simulink model "CRITIS_1_full"  (R2022b)
settings: Solver=VariableStepAuto  StartTime=0.0  StopTime=7  RelTol=1e-3
(part 12 of 13)

== system CRITIS_1_full/TELCOMMUNICATIONS1/delay ==
  in : Inport
  Clock : Clock
  Constant17 : Constant  Value=output
  Switch : Switch  Criteria=u2 > Threshold  Threshold=delay  SaturateOnIntegerOverflow=off  InputSameDT=off
  out : Outport
  wires:
  Switch/1 -> out/1
  Constant17/1 -> Switch/3
  in/1 -> Switch/1
  Clock/1 -> Switch/2

== system CRITIS_1_full/TELCOMMUNICATIONS1/delay1 ==
  in : Inport
  Clock : Clock
  Constant17 : Constant  Value=output
  Switch : Switch  Criteria=u2 > Threshold  Threshold=delay  SaturateOnIntegerOverflow=off  InputSameDT=off
  out : Outport
  wires:
  Switch/1 -> out/1
  Constant17/1 -> Switch/3
  in/1 -> Switch/1
  Clock/1 -> Switch/2

== system CRITIS_1_full/TELCOMMUNICATIONS2/Subsystem1 ==
  servizio : Inport
  Constant : Constant  Value=operation1
  Constant2 : Constant  Value=consumed1
  Constant6 : Constant  Value=operation2
  Constant7 : Constant  Value=num_serv
  Constant9 : Constant  Value=out_service
  Display : Display
  Display1 : Display
  MATLAB Function2 : MATLAB Function  TreatAsAtomicUnit=on
  EXT : Outport
  EXT_V : Outport  Port=2
  wires:
  Constant7/1 -> MATLAB Function2/5(num_serv)
  Constant9/1 -> MATLAB Function2/6(out_service)
  servizio/1 -> MATLAB Function2/1(servizio)
  Constant/1 -> Display/1, MATLAB Function2/3(operation1)
  Constant6/1 -> Display1/1, MATLAB Function2/4(operation2)
  MATLAB Function2/1(se) -> EXT/1
  MATLAB Function2/2(se_vect) -> EXT_V/1
  Constant2/1 -> MATLAB Function2/2(consumed)

== system CRITIS_1_full/TELCOMMUNICATIONS2/Subsystem3 ==
  servizio : Inport
  Constant : Constant  Value=operation1
  Constant2 : Constant  Value=consumed1
  Constant6 : Constant  Value=operation2
  Constant7 : Constant  Value=num_serv
  Constant9 : Constant  Value=out_service
  Display : Display
  Display1 : Display
  MATLAB Function2 : MATLAB Function  TreatAsAtomicUnit=on
  EXT : Outport
  EXT_V : Outport  Port=2
  wires:
  Constant7/1 -> MATLAB Function2/5(num_serv)
  Constant9/1 -> MATLAB Function2/6(out_service)
  servizio/1 -> MATLAB Function2/1(servizio)
  Constant/1 -> Display/1, MATLAB Function2/3(operation1)
  Constant6/1 -> Display1/1, MATLAB Function2/4(operation2)
  MATLAB Function2/1(se) -> EXT/1
  MATLAB Function2/2(se_vect) -> EXT_V/1
  Constant2/1 -> MATLAB Function2/2(consumed)

== system CRITIS_1_full/TELCOMMUNICATIONS2/Subsystem5 ==
  servizio : Inport
  Constant : Constant  Value=operation1
  Constant2 : Constant  Value=consumed1
  Constant6 : Constant  Value=operation2
  Constant7 : Constant  Value=num_serv
  Constant9 : Constant  Value=out_service
  Display : Display
  Display1 : Display
  MATLAB Function2 : MATLAB Function  TreatAsAtomicUnit=on
  EXT : Outport
  EXT_V : Outport  Port=2
  wires:
  Constant7/1 -> MATLAB Function2/5(num_serv)
  Constant9/1 -> MATLAB Function2/6(out_service)
  servizio/1 -> MATLAB Function2/1(servizio)
  Constant/1 -> Display/1, MATLAB Function2/3(operation1)
  Constant6/1 -> Display1/1, MATLAB Function2/4(operation2)
  MATLAB Function2/1(se) -> EXT/1
  MATLAB Function2/2(se_vect) -> EXT_V/1
  Constant2/1 -> MATLAB Function2/2(consumed)

== system CRITIS_1_full/TELCOMMUNICATIONS2/Subsystem6 ==
  servizio : Inport
  Constant : Constant  Value=operation1
  Constant2 : Constant  Value=consumed1
  Constant6 : Constant  Value=operation2
  Constant7 : Constant  Value=num_serv
  Constant9 : Constant  Value=out_service
  MATLAB Function2 : MATLAB Function  TreatAsAtomicUnit=on
  EXT : Outport
  EXT_V : Outport  Port=2
  wires:
  Constant7/1 -> MATLAB Function2/5(num_serv)
  Constant9/1 -> MATLAB Function2/6(out_service)
  servizio/1 -> MATLAB Function2/1(servizio)
  Constant/1 -> MATLAB Function2/3(operation1)
  Constant6/1 -> MATLAB Function2/4(operation2)
  MATLAB Function2/1(se) -> EXT/1
  MATLAB Function2/2(se_vect) -> EXT_V/1
  Constant2/1 -> MATLAB Function2/2(consumed)

== system CRITIS_1_full/TELCOMMUNICATIONS2/Subsystem7 ==
  servizio : Inport
  Constant : Constant  Value=operation1
  Constant2 : Constant  Value=consumed1
  Constant6 : Constant  Value=operation2
  Constant7 : Constant  Value=num_serv
  Constant9 : Constant  Value=out_service
  MATLAB Function2 : MATLAB Function  TreatAsAtomicUnit=on
  EXT : Outport
  EXT_V : Outport  Port=2
  wires:
  Constant7/1 -> MATLAB Function2/5(num_serv)
  Constant9/1 -> MATLAB Function2/6(out_service)
  servizio/1 -> MATLAB Function2/1(servizio)
  Constant/1 -> MATLAB Function2/3(operation1)
  Constant6/1 -> MATLAB Function2/4(operation2)
  MATLAB Function2/1(se) -> EXT/1
  MATLAB Function2/2(se_vect) -> EXT_V/1
  Constant2/1 -> MATLAB Function2/2(consumed)

== system CRITIS_1_full/TELCOMMUNICATIONS2/delay ==
  in : Inport
  Clock : Clock
  Constant17 : Constant  Value=output
  Switch : Switch  Criteria=u2 > Threshold  Threshold=delay  SaturateOnIntegerOverflow=off  InputSameDT=off
  out : Outport
  wires:
  Switch/1 -> out/1
  Constant17/1 -> Switch/3
  in/1 -> Switch/1
  Clock/1 -> Switch/2

== system CRITIS_1_full/TELCOMMUNICATIONS2/delay1 ==
  in : Inport
  Clock : Clock
  Constant17 : Constant  Value=output
  Switch : Switch  Criteria=u2 > Threshold  Threshold=delay  SaturateOnIntegerOverflow=off  InputSameDT=off
  out : Outport
  wires:
  Switch/1 -> out/1
  Constant17/1 -> Switch/3
  in/1 -> Switch/1
  Clock/1 -> Switch/2

== matlab function CRITIS_1_full/AIR TRANSPORTATION/ADR_Physical ==
  data: N1 input; Physical output; N2 input
function Physical = f(N1,N2)

Physical = min([N1 N2]);

== matlab function CRITIS_1_full/BANK 1/BANK1_Physical ==
  data: N1 input; Physical output
function Physical = f(N1)

Physical = min([N1]);

== matlab function CRITIS_1_full/TELCOMMUNICATIONS2/Subsystem6/MATLAB Function2 ==
  data: se output double size=1; se_vect output; servizio input; consumed input; operation1 input; operation2 input; num_serv input; out_service input; Service_Fault output
function [se,se_vect,Service_Fault] = Dep(servizio,consumed,operation1,operation2,num_serv,out_service)

Service_Fault=zeros(1,5);

for i=1:num_serv

    if operation1==1 % AND
        
        Service_Fault(i)=max(abs(consumed(:,i).*servizio(:,i)-consumed(:,i)));
      
    else % OR
        
        Service_Fault(i)=1-max(abs(consumed(:,i).*servizio(:,i)));
    end
    
end


se=1-Service_Fault(1);

if num_serv>1
    for i=2:num_serv

      if operation2==1 % AND
        se=min(se,1-Service_Fault(i));
      else % OR
        se=max(se,1-Service_Fault(i));
      end

    end
end

se_vect=zeros(1,20);
if out_service>1
    se_vect(out_service-1)=se;
end

== matlab function CRITIS_1_full/TELCOMMUNICATIONS2/Subsystem7/MATLAB Function2 ==
  data: se output double size=1; se_vect output; servizio input; consumed input; operation1 input; operation2 input; num_serv input; out_service input; Service_Fault output
function [se,se_vect,Service_Fault] = Dep(servizio,consumed,operation1,operation2,num_serv,out_service)

Service_Fault=zeros(1,5);

for i=1:num_serv

    if operation1==1 % AND
        
        Service_Fault(i)=max(abs(consumed(:,i).*servizio(:,i)-consumed(:,i)));
      
    else % OR
        
        Service_Fault(i)=1-max(abs(consumed(:,i).*servizio(:,i)));
    end
    
end


se=1-Service_Fault(1);

if num_serv>1
    for i=2:num_serv

      if operation2==1 % AND
        se=min(se,1-Service_Fault(i));
      else % OR
        se=max(se,1-Service_Fault(i));
      end

    end
end

se_vect=zeros(1,20);
if out_service>1
    se_vect(out_service-1)=se;
end

== matlab function CRITIS_1_full/ENERGY PROVIDER 1/Subsystem3/MATLAB Function2 ==
  data: se output double size=1; se_vect output; servizio input; consumed input; operation1 input; operation2 input; num_serv input; out_service input
function [se,se_vect] = Dep(servizio,consumed,operation1,operation2,num_serv,out_service)

Service_Fault=zeros(1,5);

for i=1:num_serv

    if operation1==1 % AND
        
        Service_Fault(i)=max(abs(consumed(i,:).*servizio(i,:)-consumed(i,:)));
    else % OR
        
        Service_Fault(i)=1-max(abs(consumed(i,:).*servizio(i,:)));
    end
    
end


se=1-Service_Fault(1);

if num_serv>1
    for i=2:num_serv

      if operation2==1 % AND
        se=min(se,1-Service_Fault(i));
      else % OR
        se=max(se,1-Service_Fault(i));
      end

    end
end

se_vect=zeros(1,20);
if out_service>1
    se_vect(out_service-1)=se;
end

== matlab function CRITIS_1_full/TELCOMMUNICATIONS1/Subsystem3/MATLAB Function2 ==
  data: se output double size=1; se_vect output; servizio input; consumed input; operation1 input; operation2 input; num_serv input; out_service input
function [se,se_vect] = Dep(servizio,consumed,operation1,operation2,num_serv,out_service)

Service_Fault=zeros(1,5);

for i=1:num_serv

    if operation1==1 % AND
        
        Service_Fault(i)=max(abs(consumed(i,:).*servizio(i,:)-consumed(i,:)));
    else % OR
        
        Service_Fault(i)=1-max(abs(consumed(i,:).*servizio(i,:)));
    end
    
end


se=1-Service_Fault(1);

if num_serv>1
    for i=2:num_serv

      if operation2==1 % AND
        se=min(se,1-Service_Fault(i));
      else % OR
        se=max(se,1-Service_Fault(i));
      end

    end
end

se_vect=zeros(1,20);
if out_service>1
    se_vect(out_service-1)=se;
end

== matlab function CRITIS_1_full/TELCOMMUNICATIONS1/Subsystem1/MATLAB Function2 ==
  data: se output double size=1; se_vect output; servizio input; consumed input; operation1 input; operation2 input; num_serv input; out_service input
function [se,se_vect] = Dep(servizio,consumed,operation1,operation2,num_serv,out_service)

Service_Fault=zeros(1,5);

for i=1:num_serv

    if operation1==1 % AND
        
        Service_Fault(i)=max(abs(consumed(i,:).*servizio(i,:)-consumed(i,:)));
    else % OR
        
        Service_Fault(i)=1-max(abs(consumed(i,:).*servizio(i,:)));
    end
    
end


se=1-Service_Fault(1);

if num_serv>1
    for i=2:num_serv

      if operation2==1 % AND
        se=min(se,1-Service_Fault(i));
      else % OR
        se=max(se,1-Service_Fault(i));
      end

    end
end

se_vect=zeros(1,20);
if out_service>1
    se_vect(out_service-1)=se;
end

== matlab function CRITIS_1_full/TELCOMMUNICATIONS1/Subsystem5/MATLAB Function2 ==
  data: se output double size=1; se_vect output; servizio input; consumed input; operation1 input; operation2 input; num_serv input; out_service input
function [se,se_vect] = Dep(servizio,consumed,operation1,operation2,num_serv,out_service)

Service_Fault=zeros(1,5);

for i=1:num_serv

    if operation1==1 % AND
        
        Service_Fault(i)=max(abs(consumed(i,:).*servizio(i,:)-consumed(i,:)));
    else % OR
        
        Service_Fault(i)=1-max(abs(consumed(i,:).*servizio(i,:)));
    end
    
end


se=1-Service_Fault(1);

if num_serv>1
    for i=2:num_serv

      if operation2==1 % AND
        se=min(se,1-Service_Fault(i));
      else % OR
        se=max(se,1-Service_Fault(i));
      end

    end
end

se_vect=zeros(1,20);
if out_service>1
    se_vect(out_service-1)=se;
end

== matlab function CRITIS_1_full/ENERGY PROVIDER 2/Subsystem9/MATLAB Function2 ==
  data: se output double size=1; se_vect output; servizio input; consumed input; operation1 input; operation2 input; num_serv input; out_service input; Service_Fault output
function [se,se_vect,Service_Fault] = Dep(servizio,consumed,operation1,operation2,num_serv,out_service)

Service_Fault=zeros(1,5);

for i=1:num_serv

    if operation1==1 % AND
        
        Service_Fault(i)=max(abs(consumed(:,i).*servizio(:,i)-consumed(:,i)));
      
    else % OR
        
        Service_Fault(i)=1-max(abs(consumed(:,i).*servizio(:,i)));
    end
    
end


se=1-Service_Fault(1);

if num_serv>1
    for i=2:num_serv

      if operation2==1 % AND
        se=min(se,1-Service_Fault(i));
      else % OR
        se=max(se,1-Service_Fault(i));
      end

    end
end

se_vect=zeros(1,20);
if out_service>1
    se_vect(out_service-1)=se;
end

== matlab function CRITIS_1_full/TELCOMMUNICATIONS1/Subsystem10/MATLAB Function2 ==
  data: se output double size=1; se_vect output; servizio input; consumed input; operation1 input; operation2 input; num_serv input; out_service input; Service_Fault output
function [se,se_vect,Service_Fault] = Dep(servizio,consumed,operation1,operation2,num_serv,out_service)

Service_Fault=zeros(1,5);

for i=1:num_serv

    if operation1==1 % AND
        
        Service_Fault(i)=max(abs(consumed(:,i).*servizio(:,i)-consumed(:,i)));
      
    else % OR
        
        Service_Fault(i)=1-max(abs(consumed(:,i).*servizio(:,i)));
    end
    
end


se=1-Service_Fault(1);

if num_serv>1
    for i=2:num_serv

      if operation2==1 % AND
        se=min(se,1-Service_Fault(i));
      else % OR
        se=max(se,1-Service_Fault(i));
      end

    end
end

se_vect=zeros(1,20);
if out_service>1
    se_vect(out_service-1)=se;
end

== matlab function CRITIS_1_full/AIR TRANSPORTATION/Subsystem10/MATLAB Function2 ==
  data: se output double size=1; se_vect output; servizio input; consumed input; operation1 input; operation2 input; num_serv input; out_service input; Service_Fault output
function [se,se_vect,Service_Fault] = Dep(servizio,consumed,operation1,operation2,num_serv,out_service)

Service_Fault=zeros(1,5);

for i=1:num_serv

    if operation1==1 % AND
        
        Service_Fault(i)=max(abs(consumed(:,i).*servizio(:,i)-consumed(:,i)));
      
    else % OR
        
        Service_Fault(i)=1-max(abs(consumed(:,i).*servizio(:,i)));
    end
    
end


se=1-Service_Fault(1);

if num_serv>1
    for i=2:num_serv

      if operation2==1 % AND
        se=min(se,1-Service_Fault(i));
      else % OR
        se=max(se,1-Service_Fault(i));
      end

    end
end

se_vect=zeros(1,20);
if out_service>1
    se_vect(out_service-1)=se;
end

== matlab function CRITIS_1_full/ENERGY PROVIDER 2/Subsystem1/MATLAB Function2 ==
  data: se output double size=1; se_vect output; servizio input; consumed input; operation1 input; operation2 input; num_serv input; out_service input; Service_Fault output
function [se,se_vect,Service_Fault] = Dep(servizio,consumed,operation1,operation2,num_serv,out_service)

Service_Fault=zeros(1,5);

for i=1:num_serv

    if operation1==1 % AND
        
        Service_Fault(i)=max(abs(consumed(:,i).*servizio(:,i)-consumed(:,i)));
      
    else % OR
        
        Service_Fault(i)=1-max(abs(consumed(:,i).*servizio(:,i)));
    end
    
end


se=1-Service_Fault(1);

if num_serv>1
    for i=2:num_serv

      if operation2==1 % AND
        se=min(se,1-Service_Fault(i));
      else % OR
        se=max(se,1-Service_Fault(i));
      end

    end
end

se_vect=zeros(1,20);
if out_service>1
    se_vect(out_service-1)=se;
end

== matlab function CRITIS_1_full/mean 1 ==
  data: u input; y output
function y = fcn(u)

y=[0 0];
n=length(u)/2;
y(1) = sum(u(1:2:end))/n;
y(2) = sum(u(2:2:end))/n;

== matlab function CRITIS_1_full/ENERGY PROVIDER 2/Subsystem2/MATLAB Function2 ==
  data: se output double size=1; se_vect output; servizio input; consumed input; operation1 input; operation2 input; num_serv input; out_service input; Service_Fault output
function [se,se_vect,Service_Fault] = Dep(servizio,consumed,operation1,operation2,num_serv,out_service)

Service_Fault=zeros(1,5);

for i=1:num_serv

    if operation1==1 % AND
        
        Service_Fault(i)=max(abs(consumed(:,i).*servizio(:,i)-consumed(:,i)));
      
    else % OR
        
        Service_Fault(i)=1-max(abs(consumed(:,i).*servizio(:,i)));
    end
    
end


se=1-Service_Fault(1);

if num_serv>1
    for i=2:num_serv

      if operation2==1 % AND
        se=min(se,1-Service_Fault(i));
      else % OR
        se=max(se,1-Service_Fault(i));
      end

    end
end

se_vect=zeros(1,20);
if out_service>1
    se_vect(out_service-1)=se;
end

== matlab function CRITIS_1_full/ENERGY PROVIDER 2/Subsystem4/MATLAB Function2 ==
  data: se output double size=1; se_vect output; servizio input; consumed input; operation1 input; operation2 input; num_serv input; out_service input; Service_Fault output
function [se,se_vect,Service_Fault] = Dep(servizio,consumed,operation1,operation2,num_serv,out_service)

Service_Fault=zeros(1,5);

for i=1:num_serv

    if operation1==1 % AND
        
        Service_Fault(i)=max(abs(consumed(:,i).*servizio(:,i)-consumed(:,i)));
      
    else % OR
        
        Service_Fault(i)=1-max(abs(consumed(:,i).*servizio(:,i)));
    end
    
end


se=1-Service_Fault(1);

if num_serv>1
    for i=2:num_serv

      if operation2==1 % AND
        se=min(se,1-Service_Fault(i));
      else % OR
        se=max(se,1-Service_Fault(i));
      end

    end
end

se_vect=zeros(1,20);
if out_service>1
    se_vect(out_service-1)=se;
end

== matlab function CRITIS_1_full/AIR TRANSPORTATION/Subsystem3/MATLAB Function2 ==
  data: se output double size=1; se_vect output; servizio input; consumed input; operation1 input; operation2 input; num_serv input; out_service input
function [se,se_vect] = Dep(servizio,consumed,operation1,operation2,num_serv,out_service)

Service_Fault=zeros(1,5);

for i=1:num_serv

    if operation1==1 % AND
        
        Service_Fault(i)=max(abs(consumed(i,:).*servizio(i,:)-consumed(i,:)));
    else % OR
        
        Service_Fault(i)=1-max(abs(consumed(i,:).*servizio(i,:)));
    end
    
end


se=1-Service_Fault(1);

if num_serv>1
    for i=2:num_serv

      if operation2==1 % AND
        se=min(se,1-Service_Fault(i));
      else % OR
        se=max(se,1-Service_Fault(i));
      end

    end
end

se_vect=zeros(1,20);
if out_service>1
    se_vect(out_service-1)=se;
end

== matlab function CRITIS_1_full/AIR TRANSPORTATION/Subsystem1/MATLAB Function2 ==
  data: se output double size=1; se_vect output; servizio input; consumed input; operation1 input; operation2 input; num_serv input; out_service input
function [se,se_vect] = Dep(servizio,consumed,operation1,operation2,num_serv,out_service)

Service_Fault=zeros(1,5);

for i=1:num_serv

    if operation1==1 % AND
        
        Service_Fault(i)=max(abs(consumed(i,:).*servizio(i,:)-consumed(i,:)));
    else % OR
        
        Service_Fault(i)=1-max(abs(consumed(i,:).*servizio(i,:)));
    end
    
end


se=1-Service_Fault(1);

if num_serv>1
    for i=2:num_serv

      if operation2==1 % AND
        se=min(se,1-Service_Fault(i));
      else % OR
        se=max(se,1-Service_Fault(i));
      end

    end
end

se_vect=zeros(1,20);
if out_service>1
    se_vect(out_service-1)=se;
end

== matlab function CRITIS_1_full/ENERGY PROVIDER 1/Subsystem10/MATLAB Function2 ==
  data: se output double size=1; se_vect output; servizio input; consumed input; operation1 input; operation2 input; num_serv input; out_service input; Service_Fault output
function [se,se_vect,Service_Fault] = Dep(servizio,consumed,operation1,operation2,num_serv,out_service)

Service_Fault=zeros(1,5);

for i=1:num_serv

    if operation1==1 % AND
        
        Service_Fault(i)=max(abs(consumed(:,i).*servizio(:,i)-consumed(:,i)));
      
    else % OR
        
        Service_Fault(i)=1-max(abs(consumed(:,i).*servizio(:,i)));
    end
    
end


se=1-Service_Fault(1);

if num_serv>1
    for i=2:num_serv

      if operation2==1 % AND
        se=min(se,1-Service_Fault(i));
      else % OR
        se=max(se,1-Service_Fault(i));
      end

    end
end

se_vect=zeros(1,20);
if out_service>1
    se_vect(out_service-1)=se;
end

== matlab function CRITIS_1_full/mean 2 ==
  data: u input; y output
function y = fcn(u)

y=[0 0];
n=length(u)/2;
y(1) = sum(u(1:2:end))/n;
y(2) = sum(u(2:2:end))/n;

== matlab function CRITIS_1_full/AIR TRANSPORTATION/Subsystem4/MATLAB Function2 ==
  data: se output double size=1; se_vect output; servizio input; consumed input; operation1 input; operation2 input; num_serv input; out_service input
function [se,se_vect] = Dep(servizio,consumed,operation1,operation2,num_serv,out_service)

Service_Fault=zeros(1,5);

for i=1:num_serv

    if operation1==1 % AND
        
        Service_Fault(i)=max(abs(consumed(i,:).*servizio(i,:)-consumed(i,:)));
    else % OR
        
        Service_Fault(i)=1-max(abs(consumed(i,:).*servizio(i,:)));
    end
    
end


se=1-Service_Fault(1);

if num_serv>1
    for i=2:num_serv

      if operation2==1 % AND
        se=min(se,1-Service_Fault(i));
      else % OR
        se=max(se,1-Service_Fault(i));
      end

    end
end

se_vect=zeros(1,20);
if out_service>1
    se_vect(out_service-1)=se;
end

== matlab function CRITIS_1_full/AIR TRANSPORTATION/Subsystem5/MATLAB Function2 ==
  data: se output double size=1; se_vect output; servizio input; consumed input; operation1 input; operation2 input; num_serv input; out_service input
function [se,se_vect] = Dep(servizio,consumed,operation1,operation2,num_serv,out_service)

Service_Fault=zeros(1,5);

for i=1:num_serv

    if operation1==1 % AND
        
        Service_Fault(i)=max(abs(consumed(i,:).*servizio(i,:)-consumed(i,:)));
    else % OR
        
        Service_Fault(i)=1-max(abs(consumed(i,:).*servizio(i,:)));
    end
    
end


se=1-Service_Fault(1);

if num_serv>1
    for i=2:num_serv

      if operation2==1 % AND
        se=min(se,1-Service_Fault(i));
      else % OR
        se=max(se,1-Service_Fault(i));
      end

    end
end

se_vect=zeros(1,20);
if out_service>1
    se_vect(out_service-1)=se;
end

== matlab function CRITIS_1_full/AIR TRANSPORTATION/Subsystem6/MATLAB Function2 ==
  data: se output double size=1; se_vect output; servizio input; consumed input; operation1 input; operation2 input; num_serv input; out_service input
function [se,se_vect] = Dep(servizio,consumed,operation1,operation2,num_serv,out_service)

Service_Fault=zeros(1,5);

for i=1:num_serv

    if operation1==1 % AND
        
        Service_Fault(i)=max(abs(consumed(i,:).*servizio(i,:)-consumed(i,:)));
    else % OR
        
        Service_Fault(i)=1-max(abs(consumed(i,:).*servizio(i,:)));
    end
    
end


se=1-Service_Fault(1);

if num_serv>1
    for i=2:num_serv

      if operation2==1 % AND
        se=min(se,1-Service_Fault(i));
      else % OR
        se=max(se,1-Service_Fault(i));
      end

    end
end

se_vect=zeros(1,20);
if out_service>1
    se_vect(out_service-1)=se;
end

== matlab function CRITIS_1_full/AIR TRANSPORTATION/Subsystem7/MATLAB Function2 ==
  data: se output double size=1; se_vect output; servizio input; consumed input; operation1 input; operation2 input; num_serv input; out_service input
function [se,se_vect] = Dep(servizio,consumed,operation1,operation2,num_serv,out_service)

Service_Fault=zeros(1,5);

for i=1:num_serv

    if operation1==1 % AND
        
        Service_Fault(i)=max(abs(consumed(i,:).*servizio(i,:)-consumed(i,:)));
    else % OR
        
        Service_Fault(i)=1-max(abs(consumed(i,:).*servizio(i,:)));
    end
    
end


se=1-Service_Fault(1);

if num_serv>1
    for i=2:num_serv

      if operation2==1 % AND
        se=min(se,1-Service_Fault(i));
      else % OR
        se=max(se,1-Service_Fault(i));
      end

    end
end

se_vect=zeros(1,20);
if out_service>1
    se_vect(out_service-1)=se;
end

== matlab function CRITIS_1_full/AIR TRANSPORTATION/Subsystem8/MATLAB Function2 ==
  data: se output double size=1; se_vect output; servizio input; consumed input; operation1 input; operation2 input; num_serv input; out_service input
function [se,se_vect] = Dep(servizio,consumed,operation1,operation2,num_serv,out_service)

Service_Fault=zeros(1,5);

for i=1:num_serv

    if operation1==1 % AND
        
        Service_Fault(i)=max(abs(consumed(i,:).*servizio(i,:)-consumed(i,:)));
    else % OR
        
        Service_Fault(i)=1-max(abs(consumed(i,:).*servizio(i,:)));
    end
    
end


se=1-Service_Fault(1);

if num_serv>1
    for i=2:num_serv

      if operation2==1 % AND
        se=min(se,1-Service_Fault(i));
      else % OR
        se=max(se,1-Service_Fault(i));
      end

    end
end

se_vect=zeros(1,20);
if out_service>1
    se_vect(out_service-1)=se;
end

== matlab function CRITIS_1_full/mean 3 ==
  data: u input; y output
function y = fcn(u)

y=[0 0];
n=length(u)/2;
y(1) = sum(u(1:2:end))/n;
y(2) = sum(u(2:2:end))/n;

== matlab function CRITIS_1_full/RAILWAYS/Subsystem5/MATLAB Function2 ==
  data: se output double size=1; se_vect output; servizio input; consumed input; operation1 input; operation2 input; num_serv input; out_service input
function [se,se_vect] = Dep(servizio,consumed,operation1,operation2,num_serv,out_service)

Service_Fault=zeros(1,5);

for i=1:num_serv

    if operation1==1 % AND
        
        Service_Fault(i)=max(abs(consumed(i,:).*servizio(i,:)-consumed(i,:)));
    else % OR
        
        Service_Fault(i)=1-max(abs(consumed(i,:).*servizio(i,:)));
    end
    
end


se=1-Service_Fault(1);

if num_serv>1
    for i=2:num_serv

      if operation2==1 % AND
        se=min(se,1-Service_Fault(i));
      else % OR
        se=max(se,1-Service_Fault(i));
      end

    end
end

se_vect=zeros(1,20);
if out_service>1
    se_vect(out_service-1)=se;
end

== matlab function CRITIS_1_full/RAILWAYS/Subsystem6/MATLAB Function2 ==
  data: se output double size=1; se_vect output; servizio input; consumed input; operation1 input; operation2 input; num_serv input; out_service input
function [se,se_vect] = Dep(servizio,consumed,operation1,operation2,num_serv,out_service)

Service_Fault=zeros(1,5);

for i=1:num_serv

    if operation1==1 % AND
        
        Service_Fault(i)=max(abs(consumed(i,:).*servizio(i,:)-consumed(i,:)));
    else % OR
        
        Service_Fault(i)=1-max(abs(consumed(i,:).*servizio(i,:)));
    end
    
end


se=1-Service_Fault(1);

if num_serv>1
    for i=2:num_serv

      if operation2==1 % AND
        se=min(se,1-Service_Fault(i));
      else % OR
        se=max(se,1-Service_Fault(i));
      end

    end
end

se_vect=zeros(1,20);
if out_service>1
    se_vect(out_service-1)=se;
end

== matlab function CRITIS_1_full/RAILWAYS/Subsystem1/MATLAB Function2 ==
  data: se output double size=1; se_vect output; servizio input; consumed input; operation1 input; operation2 input; num_serv input; out_service input
function [se,se_vect] = Dep(servizio,consumed,operation1,operation2,num_serv,out_service)

Service_Fault=zeros(1,5);

for i=1:num_serv

    if operation1==1 % AND
        
        Service_Fault(i)=max(abs(consumed(i,:).*servizio(i,:)-consumed(i,:)));
    else % OR
        
        Service_Fault(i)=1-max(abs(consumed(i,:).*servizio(i,:)));
    end
    
end


se=1-Service_Fault(1);

if num_serv>1
    for i=2:num_serv

      if operation2==1 % AND
        se=min(se,1-Service_Fault(i));
      else % OR
        se=max(se,1-Service_Fault(i));
      end

    end
end

se_vect=zeros(1,20);
if out_service>1
    se_vect(out_service-1)=se;
end

== matlab function CRITIS_1_full/RAILWAYS/Subsystem2/MATLAB Function2 ==
  data: se output double size=1; se_vect output; servizio input; consumed input; operation1 input; operation2 input; num_serv input; out_service input
function [se,se_vect] = Dep(servizio,consumed,operation1,operation2,num_serv,out_service)

Service_Fault=zeros(1,5);

for i=1:num_serv

    if operation1==1 % AND
        
        Service_Fault(i)=max(abs(consumed(i,:).*servizio(i,:)-consumed(i,:)));
    else % OR
        
        Service_Fault(i)=1-max(abs(consumed(i,:).*servizio(i,:)));
    end
    
end


se=1-Service_Fault(1);

if num_serv>1
    for i=2:num_serv

      if operation2==1 % AND
        se=min(se,1-Service_Fault(i));
      else % OR
        se=max(se,1-Service_Fault(i));
      end

    end
end

se_vect=zeros(1,20);
if out_service>1
    se_vect(out_service-1)=se;
end

== matlab function CRITIS_1_full/RAILWAYS/Subsystem3/MATLAB Function2 ==
  data: se output double size=1; se_vect output; servizio input; consumed input; operation1 input; operation2 input; num_serv input; out_service input
function [se,se_vect] = Dep(servizio,consumed,operation1,operation2,num_serv,out_service)

Service_Fault=zeros(1,5);

for i=1:num_serv

    if operation1==1 % AND
        
        Service_Fault(i)=max(abs(consumed(i,:).*servizio(i,:)-consumed(i,:)));
    else % OR
        
        Service_Fault(i)=1-max(abs(consumed(i,:).*servizio(i,:)));
    end
    
end


se=1-Service_Fault(1);

if num_serv>1
    for i=2:num_serv

      if operation2==1 % AND
        se=min(se,1-Service_Fault(i));
      else % OR
        se=max(se,1-Service_Fault(i));
      end

    end
end

se_vect=zeros(1,20);
if out_service>1
    se_vect(out_service-1)=se;
end

== matlab function CRITIS_1_full/RAILWAYS/Subsystem4/MATLAB Function2 ==
  data: se output double size=1; se_vect output; servizio input; consumed input; operation1 input; operation2 input; num_serv input; out_service input
function [se,se_vect] = Dep(servizio,consumed,operation1,operation2,num_serv,out_service)

Service_Fault=zeros(1,5);

for i=1:num_serv

    if operation1==1 % AND
        
        Service_Fault(i)=max(abs(consumed(i,:).*servizio(i,:)-consumed(i,:)));
    else % OR
        
        Service_Fault(i)=1-max(abs(consumed(i,:).*servizio(i,:)));
    end
    
end


se=1-Service_Fault(1);

if num_serv>1
    for i=2:num_serv

      if operation2==1 % AND
        se=min(se,1-Service_Fault(i));
      else % OR
        se=max(se,1-Service_Fault(i));
      end

    end
end

se_vect=zeros(1,20);
if out_service>1
    se_vect(out_service-1)=se;
end

== matlab function CRITIS_1_full/mean 4 ==
  data: u input; y output
function y = fcn(u)

y=[0 0];
n=length(u)/2;
y(1) = sum(u(1:2:end))/n;
y(2) = sum(u(2:2:end))/n;

== matlab function CRITIS_1_full/RAILWAYS/Subsystem7/MATLAB Function2 ==
  data: se output double size=1; se_vect output; servizio input; consumed input; operation1 input; operation2 input; num_serv input; out_service input
function [se,se_vect] = Dep(servizio,consumed,operation1,operation2,num_serv,out_service)

Service_Fault=zeros(1,5);

for i=1:num_serv

    if operation1==1 % AND
        
        Service_Fault(i)=max(abs(consumed(i,:).*servizio(i,:)-consumed(i,:)));
    else % OR
        
        Service_Fault(i)=1-max(abs(consumed(i,:).*servizio(i,:)));
    end
    
end


se=1-Service_Fault(1);

if num_serv>1
    for i=2:num_serv

      if operation2==1 % AND
        se=min(se,1-Service_Fault(i));
      else % OR
        se=max(se,1-Service_Fault(i));
      end

    end
end

se_vect=zeros(1,20);
if out_service>1
    se_vect(out_service-1)=se;
end

== matlab function CRITIS_1_full/RAILWAYS/Subsystem8/MATLAB Function2 ==
  data: se output double size=1; se_vect output; servizio input; consumed input; operation1 input; operation2 input; num_serv input; out_service input
function [se,se_vect] = Dep(servizio,consumed,operation1,operation2,num_serv,out_service)

Service_Fault=zeros(1,5);

for i=1:num_serv

    if operation1==1 % AND
        
        Service_Fault(i)=max(abs(consumed(i,:).*servizio(i,:)-consumed(i,:)));
    else % OR
        
        Service_Fault(i)=1-max(abs(consumed(i,:).*servizio(i,:)));
    end
    
end


se=1-Service_Fault(1);

if num_serv>1
    for i=2:num_serv

      if operation2==1 % AND
        se=min(se,1-Service_Fault(i));
      else % OR
        se=max(se,1-Service_Fault(i));
      end

    end
end

se_vect=zeros(1,20);
if out_service>1
    se_vect(out_service-1)=se;
end

== matlab function CRITIS_1_full/RAILWAYS/Subsystem9/MATLAB Function2 ==
  data: se output double size=1; se_vect output; servizio input; consumed input; operation1 input; operation2 input; num_serv input; out_service input
function [se,se_vect] = Dep(servizio,consumed,operation1,operation2,num_serv,out_service)

Service_Fault=zeros(1,5);

for i=1:num_serv

    if operation1==1 % AND
        
        Service_Fault(i)=max(abs(consumed(i,:).*servizio(i,:)-consumed(i,:)));
    else % OR
        
        Service_Fault(i)=1-max(abs(consumed(i,:).*servizio(i,:)));
    end
    
end


se=1-Service_Fault(1);

if num_serv>1
    for i=2:num_serv

      if operation2==1 % AND
        se=min(se,1-Service_Fault(i));
      else % OR
        se=max(se,1-Service_Fault(i));
      end

    end
end

se_vect=zeros(1,20);
if out_service>1
    se_vect(out_service-1)=se;
end

== matlab function CRITIS_1_full/RAILWAYS/Subsystem10/MATLAB Function2 ==
  data: se output double size=1; se_vect output; servizio input; consumed input; operation1 input; operation2 input; num_serv input; out_service input
function [se,se_vect] = Dep(servizio,consumed,operation1,operation2,num_serv,out_service)

Service_Fault=zeros(1,5);

for i=1:num_serv

    if operation1==1 % AND
        
        Service_Fault(i)=max(abs(consumed(i,:).*servizio(i,:)-consumed(i,:)));
    else % OR
        
        Service_Fault(i)=1-max(abs(consumed(i,:).*servizio(i,:)));
    end
    
end


se=1-Service_Fault(1);

if num_serv>1
    for i=2:num_serv

      if operation2==1 % AND
        se=min(se,1-Service_Fault(i));
      else % OR
        se=max(se,1-Service_Fault(i));
      end

    end
end

se_vect=zeros(1,20);
if out_service>1
    se_vect(out_service-1)=se;
end

== matlab function CRITIS_1_full/DEPARTMENT OF INDUSTRIAL DEVELOPMENT/Subsystem1/MATLAB Function2 ==
  data: se output double size=1; se_vect output; servizio input; consumed input; operation1 input; operation2 input; num_serv input; out_service input
function [se,se_vect] = Dep(servizio,consumed,operation1,operation2,num_serv,out_service)

Service_Fault=zeros(1,5);

for i=1:num_serv

    if operation1==1 % AND
        
        Service_Fault(i)=max(abs(consumed(i,:).*servizio(i,:)-consumed(i,:)));
    else % OR
        
        Service_Fault(i)=1-max(abs(consumed(i,:).*servizio(i,:)));
    end
    
end


se=1-Service_Fault(1);

if num_serv>1
    for i=2:num_serv

      if operation2==1 % AND
        se=min(se,1-Service_Fault(i));
      else % OR
        se=max(se,1-Service_Fault(i));
      end

    end
end

se_vect=zeros(1,20);
if out_service>1
    se_vect(out_service-1)=se;
end

== matlab function CRITIS_1_full/RAILWAYS/RFI_Physical ==
  data: N1 input; Physical output; N2 input
function Physical = f(N1,N2)

Physical = min([N1 N2]);

== matlab function CRITIS_1_full/DEPARTMENT OF INDUSTRIAL DEVELOPMENT/Subsystem2/MATLAB Function2 ==
  data: se output double size=1; se_vect output; servizio input; consumed input; operation1 input; operation2 input; num_serv input; out_service input
function [se,se_vect] = Dep(servizio,consumed,operation1,operation2,num_serv,out_service)

Service_Fault=zeros(1,5);

for i=1:num_serv

    if operation1==1 % AND
        
        Service_Fault(i)=max(abs(consumed(i,:).*servizio(i,:)-consumed(i,:)));
    else % OR
        
        Service_Fault(i)=1-max(abs(consumed(i,:).*servizio(i,:)));
    end
    
end


se=1-Service_Fault(1);

if num_serv>1
    for i=2:num_serv

      if operation2==1 % AND
        se=min(se,1-Service_Fault(i));
      else % OR
        se=max(se,1-Service_Fault(i));
      end

    end
end

se_vect=zeros(1,20);
if out_service>1
    se_vect(out_service-1)=se;
end

== matlab function CRITIS_1_full/DEPARTMENT OF INDUSTRIAL DEVELOPMENT/Subsystem3/MATLAB Function2 ==
  data: se output double size=1; se_vect output; servizio input; consumed input; operation1 input; operation2 input; num_serv input; out_service input
function [se,se_vect] = Dep(servizio,consumed,operation1,operation2,num_serv,out_service)

Service_Fault=zeros(1,5);

for i=1:num_serv

    if operation1==1 % AND
        
        Service_Fault(i)=max(abs(consumed(i,:).*servizio(i,:)-consumed(i,:)));
    else % OR
        
        Service_Fault(i)=1-max(abs(consumed(i,:).*servizio(i,:)));
    end
    
end


se=1-Service_Fault(1);

if num_serv>1
    for i=2:num_serv

      if operation2==1 % AND
        se=min(se,1-Service_Fault(i));
      else % OR
        se=max(se,1-Service_Fault(i));
      end

    end
end

se_vect=zeros(1,20);
if out_service>1
    se_vect(out_service-1)=se;
end

== matlab function CRITIS_1_full/DEPARTMENT OF INDUSTRIAL DEVELOPMENT/Subsystem4/MATLAB Function2 ==
  data: se output double size=1; se_vect output; servizio input; consumed input; operation1 input; operation2 input; num_serv input; out_service input
function [se,se_vect] = Dep(servizio,consumed,operation1,operation2,num_serv,out_service)

Service_Fault=zeros(1,5);

for i=1:num_serv

    if operation1==1 % AND
        
        Service_Fault(i)=max(abs(consumed(i,:).*servizio(i,:)-consumed(i,:)));
    else % OR
        
        Service_Fault(i)=1-max(abs(consumed(i,:).*servizio(i,:)));
    end
    
end


se=1-Service_Fault(1);

if num_serv>1
    for i=2:num_serv

      if operation2==1 % AND
        se=min(se,1-Service_Fault(i));
      else % OR
        se=max(se,1-Service_Fault(i));
      end

    end
end

se_vect=zeros(1,20);
if out_service>1
    se_vect(out_service-1)=se;
end

== matlab function CRITIS_1_full/DEPARTMENT OF INDUSTRIAL DEVELOPMENT/Subsystem5/MATLAB Function2 ==
  data: se output double size=1; se_vect output; servizio input; consumed input; operation1 input; operation2 input; num_serv input; out_service input
function [se,se_vect] = Dep(servizio,consumed,operation1,operation2,num_serv,out_service)

Service_Fault=zeros(1,5);

for i=1:num_serv

    if operation1==1 % AND
        
        Service_Fault(i)=max(abs(consumed(i,:).*servizio(i,:)-consumed(i,:)));
    else % OR
        
        Service_Fault(i)=1-max(abs(consumed(i,:).*servizio(i,:)));
    end
    
end


se=1-Service_Fault(1);

if num_serv>1
    for i=2:num_serv

      if operation2==1 % AND
        se=min(se,1-Service_Fault(i));
      else % OR
        se=max(se,1-Service_Fault(i));
      end

    end
end

se_vect=zeros(1,20);
if out_service>1
    se_vect(out_service-1)=se;
end

== matlab function CRITIS_1_full/DEPARTMENT OF INDUSTRIAL DEVELOPMENT/Subsystem6/MATLAB Function2 ==
  data: se output double size=1; se_vect output; servizio input; consumed input; operation1 input; operation2 input; num_serv input; out_service input
function [se,se_vect] = Dep(servizio,consumed,operation1,operation2,num_serv,out_service)

Service_Fault=zeros(1,5);

for i=1:num_serv

    if operation1==1 % AND
        
        Service_Fault(i)=max(abs(consumed(i,:).*servizio(i,:)-consumed(i,:)));
    else % OR
        
        Service_Fault(i)=1-max(abs(consumed(i,:).*servizio(i,:)));
    end
    
end


se=1-Service_Fault(1);

if num_serv>1
    for i=2:num_serv

      if operation2==1 % AND
        se=min(se,1-Service_Fault(i));
      else % OR
        se=max(se,1-Service_Fault(i));
      end

    end
end

se_vect=zeros(1,20);
if out_service>1
    se_vect(out_service-1)=se;
end

== matlab function CRITIS_1_full/BANK 1/Subsystem1/MATLAB Function2 ==
  data: se output double size=1; se_vect output; servizio input; consumed input; operation1 input; operation2 input; num_serv input; out_service input
function [se,se_vect] = Dep(servizio,consumed,operation1,operation2,num_serv,out_service)

Service_Fault=zeros(1,5);

for i=1:num_serv

    if operation1==1 % AND
        
        Service_Fault(i)=max(abs(consumed(i,:).*servizio(i,:)-consumed(i,:)));
    else % OR
        
        Service_Fault(i)=1-max(abs(consumed(i,:).*servizio(i,:)));
    end
    
end


se=1-Service_Fault(1);

if num_serv>1
    for i=2:num_serv

      if operation2==1 % AND
        se=min(se,1-Service_Fault(i));
      else % OR
        se=max(se,1-Service_Fault(i));
      end

    end
end

se_vect=zeros(1,20);
if out_service>1
    se_vect(out_service-1)=se;
end

== matlab function CRITIS_1_full/ENERGY PROVIDER 2/ARETI_Physical ==
  data: N1 input; Physical output; N2 input; N3 input; N4 input
function Physical = f(N1,N2,N3,N4)

Physical = min([N1 N2 N3 N4]);

== matlab function CRITIS_1_full/BANK 1/Subsystem2/MATLAB Function2 ==
  data: se output double size=1; se_vect output; servizio input; consumed input; operation1 input; operation2 input; num_serv input; out_service input
function [se,se_vect] = Dep(servizio,consumed,operation1,operation2,num_serv,out_service)

Service_Fault=zeros(1,5);

for i=1:num_serv

    if operation1==1 % AND
        
        Service_Fault(i)=max(abs(consumed(i,:).*servizio(i,:)-consumed(i,:)));
    else % OR
        
        Service_Fault(i)=1-max(abs(consumed(i,:).*servizio(i,:)));
    end
    
end


se=1-Service_Fault(1);

if num_serv>1
    for i=2:num_serv

      if operation2==1 % AND
        se=min(se,1-Service_Fault(i));
      else % OR
        se=max(se,1-Service_Fault(i));
      end

    end
end

se_vect=zeros(1,20);
if out_service>1
    se_vect(out_service-1)=se;
end

== matlab function CRITIS_1_full/BANK 1/Subsystem3/MATLAB Function2 ==
  data: se output double size=1; se_vect output; servizio input; consumed input; operation1 input; operation2 input; num_serv input; out_service input
function [se,se_vect] = Dep(servizio,consumed,operation1,operation2,num_serv,out_service)

Service_Fault=zeros(1,5);

for i=1:num_serv

    if operation1==1 % AND
        
        Service_Fault(i)=max(abs(consumed(i,:).*servizio(i,:)-consumed(i,:)));
    else % OR
        
        Service_Fault(i)=1-max(abs(consumed(i,:).*servizio(i,:)));
    end
    
end


se=1-Service_Fault(1);

if num_serv>1
    for i=2:num_serv

      if operation2==1 % AND
        se=min(se,1-Service_Fault(i));
      else % OR
        se=max(se,1-Service_Fault(i));
      end

    end
end

se_vect=zeros(1,20);
if out_service>1
    se_vect(out_service-1)=se;
end

== matlab function CRITIS_1_full/BANK 1/Subsystem4/MATLAB Function2 ==
  data: se output double size=1; se_vect output; servizio input; consumed input; operation1 input; operation2 input; num_serv input; out_service input
function [se,se_vect] = Dep(servizio,consumed,operation1,operation2,num_serv,out_service)

Service_Fault=zeros(1,5);

for i=1:num_serv

    if operation1==1 % AND
        
        Service_Fault(i)=max(abs(consumed(i,:).*servizio(i,:)-consumed(i,:)));
    else % OR
        
        Service_Fault(i)=1-max(abs(consumed(i,:).*servizio(i,:)));
    end
    
end


se=1-Service_Fault(1);

if num_serv>1
    for i=2:num_serv

      if operation2==1 % AND
        se=min(se,1-Service_Fault(i));
      else % OR
        se=max(se,1-Service_Fault(i));
      end

    end
end

se_vect=zeros(1,20);
if out_service>1
    se_vect(out_service-1)=se;
end

== matlab function CRITIS_1_full/BANK 1/Subsystem5/MATLAB Function2 ==
  data: se output double size=1; se_vect output; servizio input; consumed input; operation1 input; operation2 input; num_serv input; out_service input
function [se,se_vect] = Dep(servizio,consumed,operation1,operation2,num_serv,out_service)

Service_Fault=zeros(1,5);

for i=1:num_serv

    if operation1==1 % AND
        
        Service_Fault(i)=max(abs(consumed(i,:).*servizio(i,:)-consumed(i,:)));
    else % OR
        
        Service_Fault(i)=1-max(abs(consumed(i,:).*servizio(i,:)));
    end
    
end


se=1-Service_Fault(1);

if num_serv>1
    for i=2:num_serv

      if operation2==1 % AND
        se=min(se,1-Service_Fault(i));
      else % OR
        se=max(se,1-Service_Fault(i));
      end

    end
end

se_vect=zeros(1,20);
if out_service>1
    se_vect(out_service-1)=se;
end

== matlab function CRITIS_1_full/BANK 1/Subsystem6/MATLAB Function2 ==
  data: se output double size=1; se_vect output; servizio input; consumed input; operation1 input; operation2 input; num_serv input; out_service input
function [se,se_vect] = Dep(servizio,consumed,operation1,operation2,num_serv,out_service)

Service_Fault=zeros(1,5);

for i=1:num_serv

    if operation1==1 % AND
        
        Service_Fault(i)=max(abs(consumed(i,:).*servizio(i,:)-consumed(i,:)));
    else % OR
        
        Service_Fault(i)=1-max(abs(consumed(i,:).*servizio(i,:)));
    end
    
end


se=1-Service_Fault(1);

if num_serv>1
    for i=2:num_serv

      if operation2==1 % AND
        se=min(se,1-Service_Fault(i));
      else % OR
        se=max(se,1-Service_Fault(i));
      end

    end
end

se_vect=zeros(1,20);
if out_service>1
    se_vect(out_service-1)=se;
end

== matlab function CRITIS_1_full/AIR TRANSPORTATION/Subsystem9/MATLAB Function2 ==
  data: se output double size=1; se_vect output; servizio input; consumed input; operation1 input; operation2 input; num_serv input; out_service input; Service_Fault output
function [se,se_vect,Service_Fault] = Dep(servizio,consumed,operation1,operation2,num_serv,out_service)

Service_Fault=zeros(1,5);

for i=1:num_serv

    if operation1==1 % AND
        
        Service_Fault(i)=max(abs(consumed(:,i).*servizio(:,i)-consumed(:,i)));
      
    else % OR
        
        Service_Fault(i)=1-max(abs(consumed(:,i).*servizio(:,i)));
    end
    
end


se=1-Service_Fault(1);

if num_serv>1
    for i=2:num_serv

      if operation2==1 % AND
        se=min(se,1-Service_Fault(i));
      else % OR
        se=max(se,1-Service_Fault(i));
      end

    end
end

se_vect=zeros(1,20);
if out_service>1
    se_vect(out_service-1)=se;
end

== matlab function CRITIS_1_full/RAILWAYS/Subsystem11/MATLAB Function2 ==
  data: se output double size=1; se_vect output; servizio input; consumed input; operation1 input; operation2 input; num_serv input; out_service input; Service_Fault output
function [se,se_vect,Service_Fault] = Dep(servizio,consumed,operation1,operation2,num_serv,out_service)

Service_Fault=zeros(1,5);

for i=1:num_serv

    if operation1==1 % AND
        
        Service_Fault(i)=max(abs(consumed(:,i).*servizio(:,i)-consumed(:,i)));
      
    else % OR
        
        Service_Fault(i)=1-max(abs(consumed(:,i).*servizio(:,i)));
    end
    
end


se=1-Service_Fault(1);

if num_serv>1
    for i=2:num_serv

      if operation2==1 % AND
        se=min(se,1-Service_Fault(i));
      else % OR
        se=max(se,1-Service_Fault(i));
      end

    end
end

se_vect=zeros(1,20);
if out_service>1
    se_vect(out_service-1)=se;
end

== matlab function CRITIS_1_full/TELCOMMUNICATIONS2/Subsystem1/MATLAB Function2 ==
  data: se output double size=1; se_vect output; servizio input; consumed input; operation1 input; operation2 input; num_serv input; out_service input
function [se,se_vect] = Dep(servizio,consumed,operation1,operation2,num_serv,out_service)

Service_Fault=zeros(1,5);

for i=1:num_serv

    if operation1==1 % AND
        
        Service_Fault(i)=max(abs(consumed(i,:).*servizio(i,:)-consumed(i,:)));
    else % OR
        
        Service_Fault(i)=1-max(abs(consumed(i,:).*servizio(i,:)));
    end
    
end


se=1-Service_Fault(1);

if num_serv>1
    for i=2:num_serv

      if operation2==1 % AND
        se=min(se,1-Service_Fault(i));
      else % OR
        se=max(se,1-Service_Fault(i));
      end

    end
end

se_vect=zeros(1,20);
if out_service>1
    se_vect(out_service-1)=se;
end

== matlab function CRITIS_1_full/ENERGY PROVIDER 1/ENEL_Physical ==
  data: N1 input; Physical output; N2 input; N3 input; N4 input
function Physical = f(N1,N2,N3,N4)

Physical=0;

Physical = min([N1 N2 N3 N4]);

== matlab function CRITIS_1_full/ENERGY PROVIDER 1/Subsystem2/MATLAB Function2 ==
  data: se output double size=1; se_vect output; servizio input; consumed input; operation1 input; operation2 input; num_serv input; out_service input; Service_Fault output
function [se,se_vect,Service_Fault] = Dep(servizio,consumed,operation1,operation2,num_serv,out_service)

Service_Fault=zeros(1,5);

for i=1:num_serv

    if operation1==1 % AND
        
        Service_Fault(i)=max(abs(consumed(:,i).*servizio(:,i)-consumed(:,i)));
      
    else % OR
        
        Service_Fault(i)=1-max(abs(consumed(:,i).*servizio(:,i)));
    end
    
end


se=1-Service_Fault(1);

if num_serv>1
    for i=2:num_serv

      if operation2==1 % AND
        se=min(se,1-Service_Fault(i));
      else % OR
        se=max(se,1-Service_Fault(i));
      end

    end
end

se_vect=zeros(1,20);
if out_service>1
    se_vect(out_service-1)=se;
end

== matlab function CRITIS_1_full/TELCOMMUNICATIONS2/Subsystem3/MATLAB Function2 ==
  data: se output double size=1; se_vect output; servizio input; consumed input; operation1 input; operation2 input; num_serv input; out_service input
function [se,se_vect] = Dep(servizio,consumed,operation1,operation2,num_serv,out_service)

Service_Fault=zeros(1,5);

for i=1:num_serv

    if operation1==1 % AND
        
        Service_Fault(i)=max(abs(consumed(i,:).*servizio(i,:)-consumed(i,:)));
    else % OR
        
        Service_Fault(i)=1-max(abs(consumed(i,:).*servizio(i,:)));
    end
    
end


se=1-Service_Fault(1);

if num_serv>1
    for i=2:num_serv

      if operation2==1 % AND
        se=min(se,1-Service_Fault(i));
      else % OR
        se=max(se,1-Service_Fault(i));
      end

    end
end

se_vect=zeros(1,20);
if out_service>1
    se_vect(out_service-1)=se;
end

== matlab function CRITIS_1_full/ENERGY PROVIDER 1/Subsystem4/MATLAB Function2 ==
  data: se output double size=1; se_vect output; servizio input; consumed input; operation1 input; operation2 input; num_serv input; out_service input; Service_Fault output
function [se,se_vect,Service_Fault] = Dep(servizio,consumed,operation1,operation2,num_serv,out_service)

Service_Fault=zeros(1,5);

for i=1:num_serv

    if operation1==1 % AND
        
        Service_Fault(i)=max(abs(consumed(:,i).*servizio(:,i)-consumed(:,i)));
      
    else % OR
        
        Service_Fault(i)=1-max(abs(consumed(:,i).*servizio(:,i)));
    end
    
end


se=1-Service_Fault(1);

if num_serv>1
    for i=2:num_serv

      if operation2==1 % AND
        se=min(se,1-Service_Fault(i));
      else % OR
        se=max(se,1-Service_Fault(i));
      end

    end
end

se_vect=zeros(1,20);
if out_service>1
    se_vect(out_service-1)=se;
end
